simulink model "Gesamtsystem_VirtuelleTestUmgebung"  (R2018b)
settings: Solver=FixedStepDiscrete  StartTime=0.0  StopTime=120  RelTol=1e-3  EnableMultiTasking=on
undefined symbols (not defined in the file): sigbuilder_block
libraries: simulink x3, dspstat3 x1
(part 2 of 2)

== stateflow chart Gesamtsystem_VirtuelleTestUmgebung/sortierer virtuelle Testumgebung/Sortieralgorithmus ==
  state setupVariable
    magacin0 = 0;
    magacin1 = 0;
    magacin2 = 0;
    magacin3 = 0;
    magacin4 = 0;
    magacin5 = 0;
    magacin6 = 0;
    magacin0_LastCube = 0;
    magacin1_LastCube = 0;
    magacin2_LastCube = 0;
    magacin3_LastCube = 0;
    magacin4_LastCube = 0;
    magacin5_LastCube = 0;
    magacin6_LastCube = 0;
    magacin = -1;
    blacks = 0;
  state cubeLoaded
    magacin = -1;
  state photoelectricBarrierActivated
  state BlueCube
    entry: magacin = findPlaceForBlue();
    colourOut = 1;
  state RedCube
    entry: magacin = findPlaceForRed();
    colourOut = 2
  state Black
    magacin = 6;
    colourOut = 3;
    position = blacks;
    blacks = blacks + 1;
  state DetectedCube
  setupVariable -> cubeLoaded : [after (3, sec)]
  (default) -> setupVariable
  DetectedCube -> cubeLoaded : [cubeFinished == 0]
  cubeLoaded -> photoelectricBarrierActivated : [photoelectricBarrier < 400]
  photoelectricBarrierActivated -> Black [order 1] : [(colour > 2150)]
  photoelectricBarrierActivated -> BlueCube [order 3] : [((colour >= 1000) && (colour <= 2150)) ]
  photoelectricBarrierActivated -> RedCube [order 2] : [(colour < 1000) && (colour > 0)]
  RedCube -> DetectedCube
  BlueCube -> DetectedCube
  Black -> DetectedCube
  data: magacinOut function_output; magacinOut function_output; colour input; magacin6 local; magacin0_LastCube local; magacin3_LastCube local; magacin2_LastCube local; magacin5_LastCube local; magacin1_LastCube local; magacin6_LastCube local; magacin4_LastCube local; magacin output; photoelectricBarrier input; magacin0 local; magacin1 local; magacin2 local; magacin3 local; magacin4 local; magacin5 local; cubeFinished input; position output; colourOut output; blacks local
  function magacinOut  = findPlaceForRed:
    | function magacinOut  = findPlaceForRed
    | 
    | if((magacin1 == 0) || ((magacin1_LastCube == 1)&& (magacin1 < 5)))
    |             magacinOut = 1;
    |             magacin1 = magacin1 + 1;
    |             magacin1_LastCube = 2;
    |             position = magacin1;
    | elseif (((magacin2_LastCube == 1) && (magacin2 < 5)))
    |             magacinOut = 2;
    |             magacin2 = magacin2 + 1; 
    |             magacin2_LastCube = 2;
    |             position = magacin2;
    | elseif (magacin0 ~= 5)
    |             magacinOut = 0;
    |             magacin0 = magacin0 + 1;
    |             magacin0_LastCube = 2;
    |             position = magacin0;
    | else
    |         if (magacin3 ~= 5)
    |                 magacinOut = 3;
    |                 magacin3 = magacin3 + 1; 
    |                 magacin3_LastCube = 2;
    |                 position = magacin3;
    |         elseif ((magacin1 <= magacin4) && (magacin1 ~= 5))
    |                 magacinOut = 1;
    |                 magacin1 = magacin1 + 1; 
    |                 magacin1_LastCube = 2;
    |                 position = magacin1;
    |         elseif (magacin1 > magacin4)
    |                 magacinOut = 4;
    |                 magacin4 = magacin4 + 1;
    |                 magacin4_lastCube = 2;
    |                 position = magacin4;
    |         elseif ((magacin2 <= magacin5) && (magacin2 ~= 5))
    |                 magacinOut = 2;
    |                 magacin2 = magacin2 + 1;
    |                 magacin2_LastCube = 2;
    |                 position = magacin2;
    |         elseif (magacin2 > magacin5)
    |                 magacinOut = 5;
    |                 magacin5 = magacin5 + 1;
    |                 magacin5_LastCube = 2;
    |                 position = magacin5;
    |         else
    |                 magacinOut = -1;
    |         end            
    | end
  function magacinOut  = findPlaceForBlue:
    | function magacinOut  = findPlaceForBlue
    | 
    | %1 ist Code for Blue, 2 is Code for Red, 3 is Code for Black, 0 is empty
    | if(magacin0 == 4)  
    |             magacinOut = 0;
    |             magacin0 = (magacin0 + 1);
    |             magacin0_LastCube = 1;
    |             position = magacin0;
    | elseif ((magacin2 == 0) || (magacin2_LastCube == 2 && magacin2 < 5))
    |             magacinOut = 2;
    |             magacin2 = magacin2 + 1; 
    |             magacin2_LastCube = 1;
    |             position = magacin2;
    | elseif ((magacin1_LastCube == 2) && (magacin1 < 5))
    |             magacinOut = 1;
    |             magacin1 = magacin1 + 1;
    |             magacin1_LastCube = 1;
    |             position = magacin1;
    | elseif (magacin3 < 5)
    |             magacinOut = 3;
    |             magacin3 = (magacin3 + 1);
    |             position = magacin3;
    | elseif (magacin4 < 5)
    |             magacinOut = 4;
    |             magacin4 = (magacin4 + 1);
    |             position = magacin4;
    | elseif (magacin5 < 5)
    |             magacinOut = 5;
    |             magacin5 = (magacin5 + 1);
    |             position = magacin5;
    | else
    |             magacinOut = -1
    | end

== stateflow chart Gesamtsystem_VirtuelleTestUmgebung/Nexonar virtuelle Testumgebung/Winkelregelungssystem (Soll-Ist-Abgleich & Ausrichtungsauswertung)/Quadrantenteiler ==
  state Quadrant_a
    entry:
    Quadrant = 0;
  state Quadrant_b
    entry:
    Quadrant = 1;
  state Start_Warten
  state Quadrant_c
    entry:
    Quadrant = 2;
  state Quadrant_d
    entry:
    Quadrant = 3;
  (junction 6) -> Quadrant_a [order 1] : [x_diff >= 0 && y_diff >= 0]
  Quadrant_a -> (junction 35)
  (junction 6) -> Quadrant_b [order 2] : [x_diff <= 0 && y_diff > 0]
  Quadrant_b -> (junction 35)
  Start_Warten -> (junction 6)
  (junction 35) -> (junction 6)
  (default) -> Start_Warten
  (junction 6) -> Quadrant_c [order 3] : [x_diff < 0 && y_diff <= 0]
  Quadrant_c -> (junction 35)
  (junction 6) -> Quadrant_d [order 4]
  Quadrant_d -> (junction 35)
  data: x_diff input; y_diff input; Quadrant output

== stateflow chart Gesamtsystem_VirtuelleTestUmgebung/Nexonar virtuelle Testumgebung/Winkelregelungssystem (Soll-Ist-Abgleich & Ausrichtungsauswertung)/Winkelausgabe fuer Ausrichtung ==
  state Ausrichtung_ohne_Aenderung
    entry:
    alpha_neu = alpha_ist;
  state Start_Warten
  state Trigonometrische_Auswertung_in_Grad_fuer_Quadrant_1_3
    entry:
    alpha_neu = round(atan(abs(x_diff)/abs(y_diff))*360/(2*pi));
  state Trigonometrische_Auswertung_in_Grad_fuer_Quadrant_0_2
    entry:
    alpha_neu = round(atan(abs(y_diff)/abs(x_diff))*360/(2*pi));
  (junction 4) -> Ausrichtung_ohne_Aenderung [order 1] : [x_diff == 0 && y_diff == 0]
  Ausrichtung_ohne_Aenderung -> (junction 65)
  Start_Warten -> (junction 4)
  (junction 65) -> (junction 4)
  (default) -> Start_Warten
  (junction 4) -> Trigonometrische_Auswertung_in_Grad_fuer_Quadrant_1_3 [order 4]
  (junction 4) -> Trigonometrische_Auswertung_in_Grad_fuer_Quadrant_0_2 [order 2] : [x_diff > 0 && y_diff >= 0]
  Trigonometrische_Auswertung_in_Grad_fuer_Quadrant_0_2 -> (junction 65)
  (junction 4) -> Trigonometrische_Auswertung_in_Grad_fuer_Quadrant_0_2 [order 3] : [x_diff < 0 && y_diff <= 0]
  Trigonometrische_Auswertung_in_Grad_fuer_Quadrant_1_3 -> (junction 65)
  data: x_diff input; y_diff input; alpha_neu output; alpha_ist input

== matlab function Gesamtsystem_VirtuelleTestUmgebung/Nexonar virtuelle Testumgebung/Positionsregelungssystem (Soll-Ist-Abgleich & PWM-Auswertung)/Betrag pwm_x ==
  settings: updateMethod=DISCRETE  sampleTime=0.01
  data: x_diff_abs input; pwm_x output; Zielradius input
function pwm_x = fcn( x_diff_abs, Zielradius)

if Zielradius < x_diff_abs && x_diff_abs < 60 + Zielradius
    pwm_x = 60;
elseif x_diff_abs <= Zielradius
    pwm_x = 0;
elseif x_diff_abs >= 100 + Zielradius
    pwm_x = 100;
else
    pwm_x = x_diff_abs;
end

== matlab function Gesamtsystem_VirtuelleTestUmgebung/Nexonar virtuelle Testumgebung/Positionsregelungssystem (Soll-Ist-Abgleich & PWM-Auswertung)/Betrag pwm_y ==
  settings: updateMethod=DISCRETE  sampleTime=0.01
  data: Zielradius input; y_diff_abs input; pwm_y output
function pwm_y = fcn(Zielradius, y_diff_abs)

if Zielradius < y_diff_abs && y_diff_abs < 60 + Zielradius
    pwm_y = 60;
elseif y_diff_abs <= Zielradius
    pwm_y = 0;
elseif y_diff_abs >= 100 + Zielradius
    pwm_y = 100;
else
    pwm_y = y_diff_abs;
end
